simulink library "ACPI_lib"  (Simulink 7.5)
settings: Solver=ode45  StartTime=0.0  StopTime=10.0  RelTol=1e-3
values from neighbouring files (symbols this model uses):
  pACCI_mV_AccPed1KickDwnLo_C = Simulink.Parameter    [ACPI_par.m]
  pACCI_mV_AccPed1KickDwnUp_C = Simulink.Parameter    [ACPI_par.m]
  pACCI_mV_AccPed2KickDwnLo_C = Simulink.Parameter    [ACPI_par.m]
  pACCI_mV_AccPed2KickDwnUp_C = Simulink.Parameter    [ACPI_par.m]
  pACPI_mV_AccPed1InitMin_C = Simulink.Parameter    [ACPI_par.m]
  pACPI_mV_AccPed1MinOfst_C = Simulink.Parameter    [ACPI_par.m]
  pACPI_mV_AccPed1Pct100_C = Simulink.Parameter    [ACPI_par.m]
  pACPI_mV_AccPed1RngMax_C = Simulink.Parameter    [ACPI_par.m]
  pACPI_mV_AccPed1RngMin_C = Simulink.Parameter    [ACPI_par.m]
  pACPI_pct_AccPedMaxSensDiff_C = Simulink.Parameter    [ACPI_par.m]
  pACPI_pct_AccPedSubVal_C = Simulink.Parameter    [ACPI_par.m]
  pACPI_pct_PlausSubValMax_C = Simulink.Parameter    [ACPI_par.m]
  pACPI_pct_PlausSubValMin_C = Simulink.Parameter    [ACPI_par.m]
  pACPI_ratio_AccPed1ToAccPed2_C = Simulink.Parameter    [ACPI_par.m]
  pACPI_ratio_AccPed2ToAccPed1_C = Simulink.Parameter    [ACPI_par.m]
  pACPI_ratio_AccPedlFac_C = Simulink.Parameter    [ACPI_par.m]
undefined symbols (not defined in the file or in its folder): FAWHmiBswErrTyp, p_bool_False_M, p_bool_True_M, pACPI_pct_AccPedVal
libraries: BaseOperationLib_Browser x44, PES_CZ_FAW x4, simulink x1
settings Model: Creator=wuaibin  LastModifiedBy=wuaibin

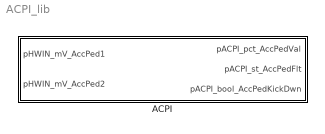
== system ACPI_lib ==
  ACPI : Subsystem  TreatAsAtomicUnit=on

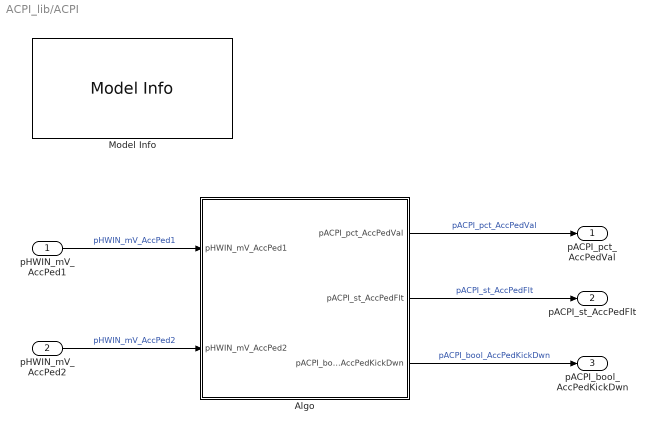
== system ACPI_lib/ACPI ==
  pHWIN_mV_AccPed1 : Inport  OutDataType=fixdt(1, 16)  OutScaling=2^0
  pHWIN_mV_AccPed2 : Inport  Port=2  OutDataType=fixdt(1, 16)  OutScaling=2^0
  Algo : Subsystem
  Model Info : simulink/Model-Wide Utilities/Model Info  SystemSampleTime=-1  InitialBlockCM=None  BlockCM=None  Frame=on  DisplayStringWithTags=Model Info\nCreated: %<Created>\nCreator: %<Creator>  HorizontalTextAlignment=Center  LeftAlignmentValue=0.5  SourceBlockDiagram=ACPI_lib  TagMaxNumber=20
  pACPI_pct_AccPedVal : Outport  OutDataType=fixdt(1, 16)  OutScaling=2^0
  pACPI_st_AccPedFlt : Outport  Port=2  OutDataType=fixdt(1, 16)  OutScaling=2^0
  pACPI_bool_AccPedKickDwn : Outport  Port=3  OutDataType=fixdt(1, 16)  OutScaling=2^0
  wires:
  Algo/2(pACPI_st_AccPedFlt) -> pACPI_st_AccPedFlt/1  "pACPI_st_AccPedFlt"
  pHWIN_mV_AccPed2/1 -> Algo/2(pHWIN_mV_AccPed2)  "pHWIN_mV_AccPed2"
  pHWIN_mV_AccPed1/1 -> Algo/1(pHWIN_mV_AccPed1)  "pHWIN_mV_AccPed1"
  Algo/1(pACPI_pct_AccPedVal) -> pACPI_pct_AccPedVal/1  "pACPI_pct_AccPedVal"
  Algo/3(pACPI_bool_AccPedKickDwn) -> pACPI_bool_AccPedKickDwn/1  "pACPI_bool_AccPedKickDwn"

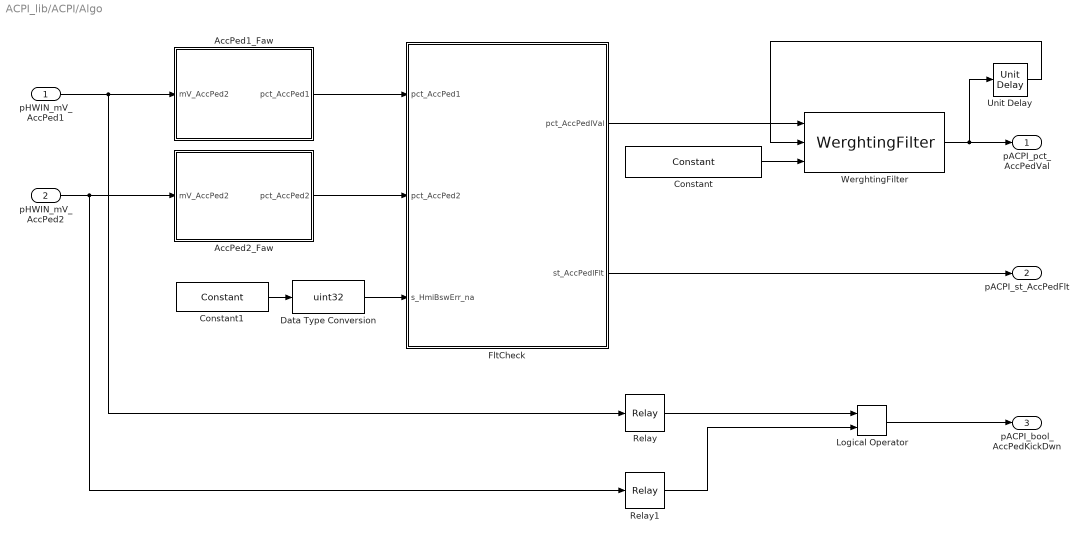
== system ACPI_lib/ACPI/Algo ==
  pHWIN_mV_AccPed1 : Inport  OutDataType=fixdt(1, 16)  OutScaling=2^0
  pHWIN_mV_AccPed2 : Inport  Port=2  OutDataType=fixdt(1, 16)  OutScaling=2^0
  AccPed1_Faw : Subsystem
  AccPed2_Faw : Subsystem
  Constant : BaseOperationLib_Browser/Sources&Sinks/Constant  Value=pACPI_ratio_AccPedlFac_C  OutMin=[]  OutMax=[]  OutDataType=fixdt(1, 16)  ConRadixGroup=Use specified scaling  OutScaling=2^0  OutDataTypeStr=Inherit: Inherit via back propagation
  Constant1 : BaseOperationLib_Browser/Sources&Sinks/Constant  Value=p_bool_False_M  OutMin=[]  OutMax=[]  OutDataType=fixdt(1, 16)  ConRadixGroup=Use specified scaling  OutScaling=2^0  OutDataTypeStr=Inherit: Inherit via back propagation
  Data Type Conversion : DataTypeConversion  OutDataTypeMode=uint32  OutDataType=fixdt(1, 16)  OutScaling=2^0  OutDataTypeStr=uint32
  FltCheck : Subsystem
  Logical Operator : BaseOperationLib_Browser/Logic Operations Changed/Logical Operator  Operator=AND  Inputs=2  AllPortsSameDT=on  OutDataTypeMode=Specify via dialog  LogicDataType=PDT_Bool  OutDataTypeStr=PDT_Bool
  Relay : BaseOperationLib_Browser/Discontinuities Changed/Relay  OnSwitchValue=pACCI_mV_AccPed1KickDwnUp_C  OffSwitchValue=pACCI_mV_AccPed1KickDwnLo_C  OnOutputValue=p_bool_True_M  OffOutputValue=p_bool_False_M  OutMin=[]  OutMax=[]  OutDataType=fixdt(1, 16)  ConRadixGroup=Use specified scaling  OutScaling=2^0  OutDataTypeStr=Inherit: Inherit via back propagation
      settings: AttributesFormatString=%<OnSwitchValue> OnOut %<OnOutputValue>\n%<OffSwitchValue> OffOut %<OffOutputValue>
  Relay1 : BaseOperationLib_Browser/Discontinuities Changed/Relay  OnSwitchValue=pACCI_mV_AccPed2KickDwnUp_C  OffSwitchValue=pACCI_mV_AccPed2KickDwnLo_C  OnOutputValue=p_bool_True_M  OffOutputValue=p_bool_False_M  OutMin=[]  OutMax=[]  OutDataType=fixdt(1, 16)  ConRadixGroup=Use specified scaling  OutScaling=2^0  OutDataTypeStr=Inherit: Inherit via back propagation
      settings: AttributesFormatString=%<OnSwitchValue> OnOut %<OnOutputValue>\n%<OffSwitchValue> OffOut %<OffOutputValue>
  Unit Delay : BaseOperationLib_Browser/Discrete Unchanged /Unit Delay  X0=0  SampleTime=-1
  WerghtingFilter : BaseOperationLib_Browser/Discontinuities Unchanged/WerghtingFilter  SystemSampleTime=-1
  pACPI_pct_AccPedVal : Outport  OutDataType=fixdt(1, 16)  OutScaling=2^0
  pACPI_st_AccPedFlt : Outport  Port=2  OutDataType=fixdt(1, 16)  OutScaling=2^0
  pACPI_bool_AccPedKickDwn : Outport  Port=3  OutDataType=fixdt(1, 16)  OutScaling=2^0
  wires:
  Data Type Conversion/1 -> FltCheck/3(s_HmiBswErr_na)
  pHWIN_mV_AccPed2/1 -> AccPed2_Faw/1(mV_AccPed2), Relay1/1
  pHWIN_mV_AccPed1/1 -> AccPed1_Faw/1(mV_AccPed2), Relay/1
  Constant1/1 -> Data Type Conversion/1
  Unit Delay/1 -> WerghtingFilter/2
  Constant/1 -> WerghtingFilter/3
  FltCheck/1(pct_AccPedlVal) -> WerghtingFilter/1
  WerghtingFilter/1 -> Unit Delay/1, pACPI_pct_AccPedVal/1
  AccPed1_Faw/1(pct_AccPed1) -> FltCheck/1(pct_AccPed1)
  AccPed2_Faw/1(pct_AccPed2) -> FltCheck/2(pct_AccPed2)
  FltCheck/2(st_AccPedlFlt) -> pACPI_st_AccPedFlt/1
  Relay/1 -> Logical Operator/1
  Logical Operator/1 -> pACPI_bool_AccPedKickDwn/1
  Relay1/1 -> Logical Operator/2

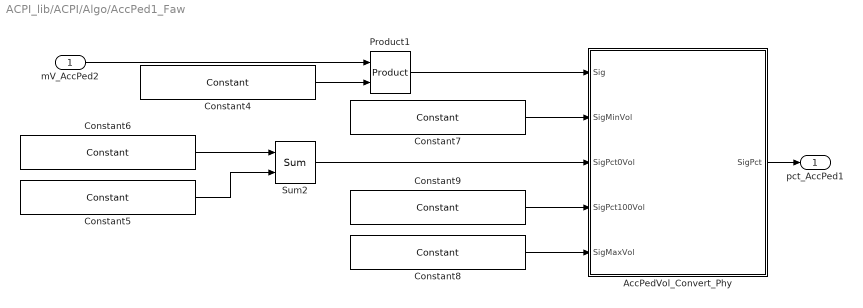
== system ACPI_lib/ACPI/Algo/AccPed1_Faw ==
  mV_AccPed2 : Inport
  AccPedVol_Convert_Phy : Stateflow chart  TreatAsAtomicUnit=on
  Constant4 : BaseOperationLib_Browser/Sources&Sinks/Constant  Value=pACPI_ratio_AccPed1ToAccPed2_C  OutMin=[]  OutMax=[]  OutDataType=fixdt(1, 16)  ConRadixGroup=Use specified scaling  OutScaling=2^0  OutDataTypeStr=Inherit: Inherit from 'Constant value'
  Constant5 : BaseOperationLib_Browser/Sources&Sinks/Constant  Value=pACPI_mV_AccPed1MinOfst_C  OutMin=[]  OutMax=[]  OutDataType=fixdt(1, 16)  ConRadixGroup=Use specified scaling  OutScaling=2^0  OutDataTypeStr=Inherit: Inherit from 'Constant value'
  Constant6 : BaseOperationLib_Browser/Sources&Sinks/Constant  Value=pACPI_mV_AccPed1InitMin_C  OutMin=[]  OutMax=[]  OutDataType=fixdt(1, 16)  ConRadixGroup=Use specified scaling  OutScaling=2^0  OutDataTypeStr=Inherit: Inherit from 'Constant value'
  Constant7 : BaseOperationLib_Browser/Sources&Sinks/Constant  Value=pACPI_mV_AccPed1RngMin_C  OutMin=[]  OutMax=[]  OutDataType=fixdt(1, 16)  ConRadixGroup=Use specified scaling  OutScaling=2^0  OutDataTypeStr=Inherit: Inherit from 'Constant value'
  Constant8 : BaseOperationLib_Browser/Sources&Sinks/Constant  Value=pACPI_mV_AccPed1RngMax_C  OutMin=[]  OutMax=[]  OutDataType=fixdt(1, 16)  ConRadixGroup=Use specified scaling  OutScaling=2^0  OutDataTypeStr=Inherit: Inherit from 'Constant value'
  Constant9 : BaseOperationLib_Browser/Sources&Sinks/Constant  Value=pACPI_mV_AccPed1Pct100_C  OutMin=[]  OutMax=[]  OutDataType=fixdt(1, 16)  ConRadixGroup=Use specified scaling  OutScaling=2^0  OutDataTypeStr=Inherit: Inherit from 'Constant value'
  Product1 : BaseOperationLib_Browser/Math Operations Changed/Product  Inputs=2  Multiplication=Element-wise(.*)  OutMin=[]  OutMax=[]  OutDataType=fixdt(1,16,0)  OutScaling=[]  OutDataTypeStr=Inherit: Inherit via back propagation  RndMeth=Zero  SaturateOnIntegerOverflow=on
  Sum2 : BaseOperationLib_Browser/Math Operations Changed/Sum  Inputs=++  InputSameDT=on  OutMin=[]  OutMax=[]  OutDataType=fixdt(1, 16)  OutScaling=2^0  SaturateOnIntegerOverflow=on
  pct_AccPed1 : Outport
  wires:
  AccPedVol_Convert_Phy/1(SigPct) -> pct_AccPed1/1
  Sum2/1 -> AccPedVol_Convert_Phy/3(SigPct0Vol)
  Constant7/1 -> AccPedVol_Convert_Phy/2(SigMinVol)
  Constant8/1 -> AccPedVol_Convert_Phy/5(SigMaxVol)
  Constant9/1 -> AccPedVol_Convert_Phy/4(SigPct100Vol)
  Constant5/1 -> Sum2/2
  Constant6/1 -> Sum2/1
  Constant4/1 -> Product1/2
  mV_AccPed2/1 -> Product1/1
  Product1/1 -> AccPedVol_Convert_Phy/1(Sig)

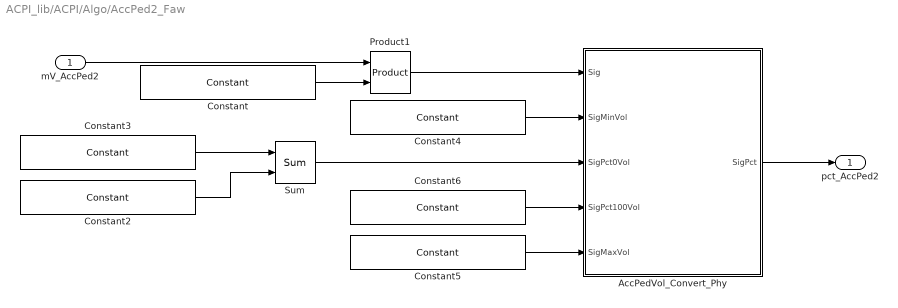
== system ACPI_lib/ACPI/Algo/AccPed2_Faw ==
  mV_AccPed2 : Inport
  AccPedVol_Convert_Phy : Stateflow chart  TreatAsAtomicUnit=on
  Constant : BaseOperationLib_Browser/Sources&Sinks/Constant  Value=pACPI_ratio_AccPed2ToAccPed1_C  OutMin=[]  OutMax=[]  OutDataType=fixdt(1, 16)  ConRadixGroup=Use specified scaling  OutScaling=2^0  OutDataTypeStr=Inherit: Inherit from 'Constant value'
  Constant2 : BaseOperationLib_Browser/Sources&Sinks/Constant  Value=pACPI_mV_AccPed1MinOfst_C  OutMin=[]  OutMax=[]  OutDataType=fixdt(1, 16)  ConRadixGroup=Use specified scaling  OutScaling=2^0  OutDataTypeStr=Inherit: Inherit from 'Constant value'
  Constant3 : BaseOperationLib_Browser/Sources&Sinks/Constant  Value=pACPI_mV_AccPed1InitMin_C  OutMin=[]  OutMax=[]  OutDataType=fixdt(1, 16)  ConRadixGroup=Use specified scaling  OutScaling=2^0  OutDataTypeStr=Inherit: Inherit from 'Constant value'
  Constant4 : BaseOperationLib_Browser/Sources&Sinks/Constant  Value=pACPI_mV_AccPed1RngMin_C  OutMin=[]  OutMax=[]  OutDataType=fixdt(1, 16)  ConRadixGroup=Use specified scaling  OutScaling=2^0  OutDataTypeStr=Inherit: Inherit from 'Constant value'
  Constant5 : BaseOperationLib_Browser/Sources&Sinks/Constant  Value=pACPI_mV_AccPed1RngMax_C  OutMin=[]  OutMax=[]  OutDataType=fixdt(1, 16)  ConRadixGroup=Use specified scaling  OutScaling=2^0  OutDataTypeStr=Inherit: Inherit from 'Constant value'
  Constant6 : BaseOperationLib_Browser/Sources&Sinks/Constant  Value=pACPI_mV_AccPed1Pct100_C  OutMin=[]  OutMax=[]  OutDataType=fixdt(1, 16)  ConRadixGroup=Use specified scaling  OutScaling=2^0  OutDataTypeStr=Inherit: Inherit from 'Constant value'
  Product1 : BaseOperationLib_Browser/Math Operations Changed/Product  Inputs=2  Multiplication=Element-wise(.*)  OutMin=[]  OutMax=[]  OutDataType=fixdt(1,16,0)  OutScaling=[]  OutDataTypeStr=Inherit: Inherit via back propagation  RndMeth=Zero  SaturateOnIntegerOverflow=on
  Sum : BaseOperationLib_Browser/Math Operations Changed/Sum  Inputs=++  InputSameDT=on  OutMin=[]  OutMax=[]  OutDataType=fixdt(1, 16)  OutScaling=2^0  SaturateOnIntegerOverflow=on
  pct_AccPed2 : Outport
  wires:
  Product1/1 -> AccPedVol_Convert_Phy/1(Sig)
  mV_AccPed2/1 -> Product1/1
  Constant/1 -> Product1/2
  AccPedVol_Convert_Phy/1(SigPct) -> pct_AccPed2/1
  Constant3/1 -> Sum/1
  Constant2/1 -> Sum/2
  Constant6/1 -> AccPedVol_Convert_Phy/4(SigPct100Vol)
  Constant5/1 -> AccPedVol_Convert_Phy/5(SigMaxVol)
  Constant4/1 -> AccPedVol_Convert_Phy/2(SigMinVol)
  Sum/1 -> AccPedVol_Convert_Phy/3(SigPct0Vol)

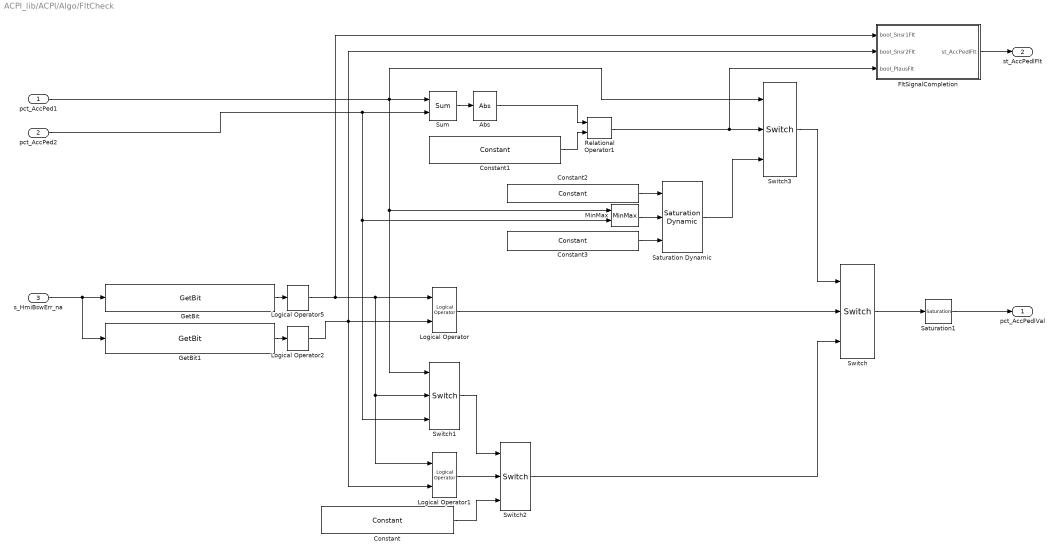
== system ACPI_lib/ACPI/Algo/FltCheck ==
  pct_AccPed1 : Inport  OutDataType=fixdt(1, 16)  OutScaling=2^0
  pct_AccPed2 : Inport  Port=2  OutDataType=fixdt(1, 16)  OutScaling=2^0
  s_HmiBswErr_na : Inport  Port=3  OutDataType=fixdt(1, 16)  OutScaling=2^0
  Abs : BaseOperationLib_Browser/Math Operations Changed/Abs  OutMax=[]  OutDataType=fixdt(1, 16)  OutScaling=2^0  SaturateOnIntegerOverflow=on
  Constant : BaseOperationLib_Browser/Sources&Sinks/Constant  Value=pACPI_pct_AccPedSubVal_C  OutMin=[]  OutMax=[]  OutDataType=fixdt(1, 16)  ConRadixGroup=Use specified scaling  OutScaling=2^0  OutDataTypeStr=Inherit: Inherit via back propagation
  Constant1 : BaseOperationLib_Browser/Sources&Sinks/Constant  Value=pACPI_pct_AccPedMaxSensDiff_C  OutMin=[]  OutMax=[]  OutDataType=fixdt(1, 16)  ConRadixGroup=Use specified scaling  OutScaling=2^0  OutDataTypeStr=Inherit: Inherit via back propagation
  Constant2 : BaseOperationLib_Browser/Sources&Sinks/Constant  Value=pACPI_pct_PlausSubValMax_C  OutMin=[]  OutMax=[]  OutDataType=fixdt(1, 16)  ConRadixGroup=Use specified scaling  OutScaling=2^0  OutDataTypeStr=Inherit: Inherit via back propagation
  Constant3 : BaseOperationLib_Browser/Sources&Sinks/Constant  Value=pACPI_pct_PlausSubValMin_C  OutMin=[]  OutMax=[]  OutDataType=fixdt(1, 16)  ConRadixGroup=Use specified scaling  OutScaling=2^0  OutDataTypeStr=Inherit: Inherit via back propagation
  FltSignalCompletion : Subsystem
  GetBit : PES_CZ_FAW/Discontinuities/GetBit  SystemSampleTime=-1  maska=uint32(FAWHmiBswErrTyp.ACCR_PEDAL_1_ERROR)
  GetBit1 : PES_CZ_FAW/Discontinuities/GetBit  SystemSampleTime=-1  maska=uint32(FAWHmiBswErrTyp.ACCR_PEDAL_2_ERROR)
  Logical Operator : BaseOperationLib_Browser/Logic Operations Changed/Logical Operator  Operator=AND  Inputs=2  AllPortsSameDT=on  OutDataTypeMode=Specify via dialog  LogicDataType=PDT_Bool  OutDataTypeStr=PDT_Bool
  Logical Operator1 : BaseOperationLib_Browser/Logic Operations Changed/Logical Operator  Operator=OR  Inputs=2  AllPortsSameDT=on  OutDataTypeMode=Specify via dialog  LogicDataType=PDT_Bool  OutDataTypeStr=PDT_Bool
  Logical Operator2 : BaseOperationLib_Browser/Logic Operations Changed/Logical Operator  Operator=NOT  Inputs=2  AllPortsSameDT=on  OutDataTypeMode=Specify via dialog  LogicDataType=PDT_Bool  OutDataTypeStr=PDT_Bool
  Logical Operator5 : BaseOperationLib_Browser/Logic Operations Changed/Logical Operator  Operator=NOT  Inputs=2  AllPortsSameDT=on  OutDataTypeMode=Specify via dialog  LogicDataType=PDT_Bool  OutDataTypeStr=PDT_Bool
  MinMax : BaseOperationLib_Browser/Math Operations Changed/MinMax  Function=min  Inputs=2  InputSameDT=on  OutMin=[]  OutMax=[]  OutDataType=fixdt(1, 16)  OutScaling=2^0  SaturateOnIntegerOverflow=on
  Relational Operator1 : BaseOperationLib_Browser/Logic Operations Changed/Relational Operator  Operator=<=  InputSameDT=on  LogicOutDataTypeMode=Specify via dialog  LogicDataType=PDT_Bool  OutDataTypeStr=PDT_Bool
  Saturation Dynamic : BaseOperationLib_Browser/Discontinuities Unchanged/Saturation Dynamic  SystemSampleTime=-1  OutMin=[]  OutMax=[]  OutDataTypeStr=Inherit: Same as second input  OutDataType=fixdt(1, 16)  OutScaling=2^-10  DoSatur=on
  Saturation1 : BaseOperationLib_Browser/Discontinuities Unchanged/Saturation  UpperLimit=pACPI_pct_AccPedVal.Max  LowerLimit=pACPI_pct_AccPedVal.Min  OutMin=[]  OutMax=[]  OutDataType=fixdt(1, 16)  OutScaling=2^0
      settings: AttributesFormatString=ULim:%<UpperLimit>\nLLim:%<LowerLimit>
  Sum : BaseOperationLib_Browser/Math Operations Changed/Sum  Inputs=+-  InputSameDT=on  OutMin=[]  OutMax=[]  OutDataType=fixdt(1, 16)  OutScaling=2^0  SaturateOnIntegerOverflow=on
  Switch{,1..3} (4 alike) : BaseOperationLib_Browser/Signal Routing Changed/Switch  Criteria=u2 ~= 0  Threshold=1  InputSameDT=on  OutMin=[]  OutMax=[]  OutDataType=fixdt(1,16,0)  OutScaling=[]  SaturateOnIntegerOverflow=on
  pct_AccPedlVal : Outport  OutDataType=fixdt(1, 16)  OutScaling=2^0
  st_AccPedlFlt : Outport  Port=2  OutDataType=fixdt(1, 16)  OutScaling=2^0
  wires:
  Constant3/1 -> Saturation Dynamic/3
  Constant2/1 -> Saturation Dynamic/1
  MinMax/1 -> Saturation Dynamic/2
  GetBit/1 -> Logical Operator5/1
  GetBit1/1 -> Logical Operator2/1
  Abs/1 -> Relational Operator1/1
  Sum/1 -> Abs/1
  Constant1/1 -> Relational Operator1/2
  pct_AccPed1/1 -> Sum/1, Switch3/1, Switch1/1, MinMax/1
  pct_AccPed2/1 -> Sum/2, Switch1/3, MinMax/2
  s_HmiBswErr_na/1 -> GetBit1/1, GetBit/1
  Switch1/1 -> Switch2/1
  Logical Operator/1 -> Switch/2
  Relational Operator1/1 -> Switch3/2, FltSignalCompletion/3(bool_PlausFlt)
  Switch3/1 -> Switch/1
  Switch/1 -> Saturation1/1
  Logical Operator1/1 -> Switch2/2
  Constant/1 -> Switch2/3
  Switch2/1 -> Switch/3
  Saturation1/1 -> pct_AccPedlVal/1
  Saturation Dynamic/1 -> Switch3/3
  FltSignalCompletion/1(st_AccPedlFlt) -> st_AccPedlFlt/1
  Logical Operator5/1 -> Switch1/2, Logical Operator1/1, Logical Operator/1, FltSignalCompletion/1(bool_Snsr1Flt)
  Logical Operator2/1 -> Logical Operator1/2, FltSignalCompletion/2(bool_Snsr2Flt), Logical Operator/2

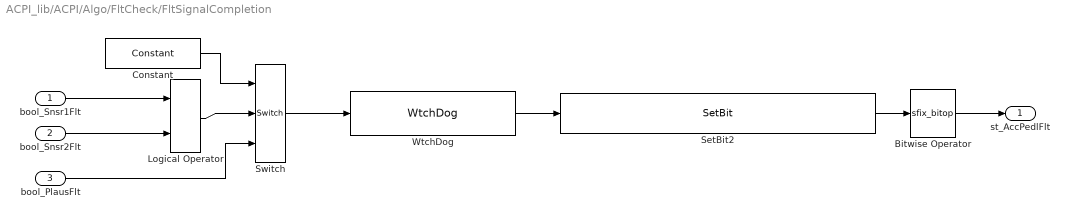
== system ACPI_lib/ACPI/Algo/FltCheck/FltSignalCompletion ==
  bool_Snsr1Flt : Inport  OutDataType=fixdt(1, 16)  OutScaling=2^0
  bool_Snsr2Flt : Inport  Port=2  OutDataType=fixdt(1, 16)  OutScaling=2^0
  bool_PlausFlt : Inport  Port=3  OutDataType=fixdt(1, 16)  OutScaling=2^0
  Bitwise Operator : S-Function  FunctionName=sfix_bitop  Parameters=UseBitMask,NumInputPorts,BitMask,BitMaskRealWorld,logicop  EnableBusSupport=off  mask(Bitwise Operator){logicop=OR, UseBitMask=off, NumInputPorts=1, BitMask=bin2dec('11011001'), BitMaskRealWorld=Stored Integer}
      mask prompts: logicop "Operator:"; UseBitMask "Use bit mask ..."; NumInputPorts "Number of input ports:"; BitMask "Bit Mask"; BitMaskRealWorld "Treat mask as:"
      mask help: Perform the specified bitwise operation on the inputs. The output data type should represent zero exactly.
      mask init:
      | str = '';
      | if UseBitMask
      |   [m,n] = size(BitMask);
      |   if ischar(BitMask)
      |     len = m;
      |     n = 1;
      |   else
      |     len = m * n;
      |   end
      |   internalBitMask = zeros(m,n);
      |   if isnumeric(BitMask)
      |     for i=1:len,
      |       internalBitMask(i) = BitMask(i);
      |     end
      |   elseif ischar(BitMask)
      |     for i=1:m,
      |       internalBitMask(i) = hex2dec(BitMask(i,:));
      |     end
      |   elseif iscell(BitMask)
      |     for i=1:len,
      |       if isnumeric( BitMask{i} )
      |         internalBitMask(i) = BitMask{i};
      |       elseif ischar( BitMask{i} )
      |         internalBitMask(i) = hex2dec(BitMask{i});
      |       else
      |         errordlg(['Data type is not supported at cell item ', num2str(i) ]);
      |       end
      |     end
      |   end
      |   BitMask = internalBitMask;
      |   for i=1:len
      |     if BitMask(i) > (2^52)-1
      |       error(DAStudio.message('Simulink:blocks:BitMaskWordLengthTooLarge')); 
      |     end
      |   end 
      |   if len == 1
      |      if BitMaskRealWorld == 1 || BitMask(1) < 0
      |        str=num2str(BitMask(1));
      |      else
      |        str=['0x',dec2hex(floor(BitMask(1)))];
      |      end
      |   else
      |      str='Masks';
      |   end
      | else
      |   BitMask = 0;
      |   str='';
      | end
      mask StyleString: popup(AND|OR|NAND|NOR|XOR|NOT),checkbox,edit,edit,popup(Real World Value|Stored Integer)
      mask CallbackString: fixptdialog(gcbh)|fixptdialog(gcbh)|||
      mask Display: fprintf(['Bitwise\n',logicop,'\n',str])
  Constant : BaseOperationLib_Browser/Sources&Sinks/Constant  Value=p_bool_True_M  OutMin=[]  OutMax=[]  OutDataType=fixdt(1, 16)  ConRadixGroup=Use specified scaling  OutScaling=2^0  OutDataTypeStr=Inherit: Inherit via back propagation
  Logical Operator : BaseOperationLib_Browser/Logic Operations Changed/Logical Operator  Operator=AND  Inputs=2  AllPortsSameDT=on  OutDataTypeMode=Specify via dialog  LogicDataType=PDT_Bool  OutDataTypeStr=PDT_Bool
  SetBit2 : PES_CZ_FAW/Discontinuities/SetBit  SystemSampleTime=-1  maska=AccrPedlFltTyp.ACCR_PEDAL_PLAUSIBILITY_ERROR
  Switch : BaseOperationLib_Browser/Signal Routing Changed/Switch  Criteria=u2 ~= 0  Threshold=1  InputSameDT=on  OutMin=[]  OutMax=[]  OutDataType=fixdt(1,16,0)  OutScaling=[]  SaturateOnIntegerOverflow=on
  WtchDog : PES_CZ_FAW/Discontinuities/WtchDog  SystemSampleTime=-1  timeoutthres=pACPI_s_AccPedTiout_C
  st_AccPedlFlt : Outport  OutDataType=fixdt(1, 16)  OutScaling=2^0
  wires:
  Switch/1 -> WtchDog/1
  Constant/1 -> Switch/1
  Logical Operator/1 -> Switch/2
  WtchDog/1 -> SetBit2/1
  SetBit2/1 -> Bitwise Operator/1
  Bitwise Operator/1 -> st_AccPedlFlt/1
  bool_Snsr1Flt/1 -> Logical Operator/1
  bool_Snsr2Flt/1 -> Logical Operator/2
  bool_PlausFlt/1 -> Switch/3

== stateflow chart ACPI/Algo/AccPed1_Faw/AccPedVol_Convert_Phy ==
  (default) -> (junction 3)
  (junction 3) -> (junction 4) [order 2]
  (junction 3) -> (junction 5) [order 1] : [Sig<SigMinVol]
  (junction 5) -> (junction 6) : {SigPct=0;}
  (junction 4) -> (junction 7) [order 1] : [Sig<SigPct0Vol]
  (junction 7) -> (junction 8) : {SigPct=0;}
  (junction 4) -> (junction 9) [order 2]
  (junction 9) -> (junction 10) [order 1] : [Sig<SigPct100Vol]
  (junction 10) -> (junction 11) : {SigPct=100*(Sig-SigPct0Vol)/(SigPct100Vol-SigPct0Vol);}
  (junction 9) -> (junction 12) [order 2]
  (junction 12) -> (junction 13) [order 1] : [Sig<SigMaxVol]
  (junction 13) -> (junction 14) : {SigPct=100;}
  (junction 12) -> (junction 15) [order 2] : {SigPct=100;}
  (junction 6) -> (junction 8)
  (junction 8) -> (junction 11)
  (junction 11) -> (junction 14)
  (junction 14) -> (junction 15)
  data: Sig input double; SigMinVol input double; SigPct0Vol input double; SigPct100Vol input double; SigMaxVol input double; SigPct output double

== stateflow chart ACPI/Algo/AccPed2_Faw/AccPedVol_Convert_Phy ==
  (default) -> (junction 41)
  (junction 41) -> (junction 42) [order 2]
  (junction 41) -> (junction 43) [order 1] : [Sig<SigMinVol]
  (junction 43) -> (junction 44) : {SigPct=0;}
  (junction 42) -> (junction 45) [order 1] : [Sig<SigPct0Vol]
  (junction 45) -> (junction 46) : {SigPct=0;}
  (junction 42) -> (junction 47) [order 2]
  (junction 47) -> (junction 48) [order 1] : [Sig<SigPct100Vol]
  (junction 48) -> (junction 49) : {SigPct=100*(Sig-SigPct0Vol)/(SigPct100Vol-SigPct0Vol);}
  (junction 47) -> (junction 50) [order 2]
  (junction 50) -> (junction 51) [order 1] : [Sig<SigMaxVol]
  (junction 51) -> (junction 52) : {SigPct=100;}
  (junction 50) -> (junction 53) [order 2] : {SigPct=100;}
  (junction 44) -> (junction 46)
  (junction 46) -> (junction 49)
  (junction 49) -> (junction 52)
  (junction 52) -> (junction 53)
  data: Sig input double; SigMinVol input double; SigPct0Vol input double; SigPct100Vol input double; SigMaxVol input double; SigPct output double
